simulink model "reference_generator"  (Simulink 8.2)
settings: Solver=FixedStepDiscrete  StartTime=0.0  StopTime=60  FixedStep=0.1  RelTol=1e-3
undefined symbols (not defined in the file or in its folder): sigbuilder_block
settings Model: Creator=ovidiua  LastModifiedBy=ovidiua
settings DataIOCC: SignalLoggingSaveFormat=Dataset
settings OptimizationCC: ExpressionDepthLimit=128
settings DebuggingCC: FcnCallInpInsideContextMsg=EnableAllAsError  StateNameClashWarn=none
settings GRTTargetCC: CombineOutputUpdateFcns=on  GRTInterface=off

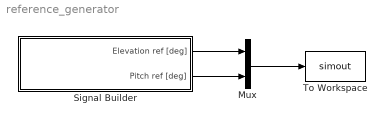
== system reference_generator ==
  Mux : Mux  Inputs=2
  Signal Builder : Subsystem  Tag=STV Subsys  LoadFcn=sigbuilder_block('load');  StartFcn=sigbuilder_block('start');  StopFcn=sigbuilder_block('stop');  ClipboardFcn=sigbuilder_block('clipboard');  mask(Sigbuilder block){}
      mask help: Simulink:masks:SigbuilderBlock_MD
      mask init:
      | if ~strcmp(get_param(bdroot(gcbh),'SimulationStatus'),'stopped') tuvar = sigbuilder_block('maskInit'); end
      settings: CopyFcn=sigbuilder_block('copy');  DeleteFcn=sigbuilder_block('delete');  ModelCloseFcn=sigbuilder_block('modelClose');  PreSaveFcn=sigbuilder_block('preSave');  PauseFcn=sigbuilder_block('pause');  ContinueFcn=sigbuilder_block('continue');  NameChangeFcn=sigbuilder_block('namechange');  OpenFcn=sigbuilder_block('open',[446.25 160.5 761.25 513.75 ]);  CloseFcn=sigbuilder_block('close');
      mask Display: plot(0, 0, 100, 100,[2, 2, 32, 32, 2], [68, 8, 8, 68, 68],[32, 2], [38, 38], [32, 19, 2],[53, 60, 44], [32, 17, 17, 2],[16, 16, 31, 31]);txt = getActiveGroup(gcbh);text(2, 100, txt,'verticalAlignment', 'top');
  To Workspace : ToWorkspace  VariableName=simout  SampleTime=-1  SaveFormat=Timeseries
  wires:
  Signal Builder/1(Elevation ref [deg]) -> Mux/1
  Signal Builder/2(Pitch ref [deg]) -> Mux/2
  Mux/1 -> To Workspace/1

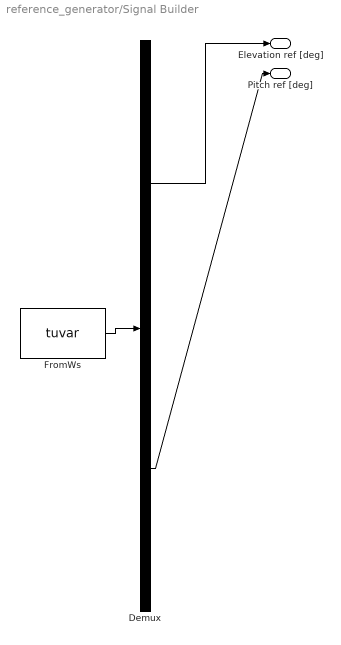
== system reference_generator/Signal Builder ==
  Demux : Demux  Tag=STV Demux  Outputs=2
  FromWs : FromWorkspace  Tag=STV FromWs  VariableName=tuvar  SampleTime=0  SigBuilderData=DataTag0  VnvData=DataTag1
      SigBuilderData=|
      | common.afterFinalStr = 'Extrapolate'
      | common.sampleTime = 0
      | dataSet.timeRange = [0 60]
      | dataSet.name = 'Group 1'
      | sbobj.Groups.Name = 'Group 1'
      | sbobj.Groups.Signals(1).Name = 'Elevation ref [deg]'
      | sbobj.Groups.Signals(1).XData = [0 10 15 40 45 50 55 60]
      | sbobj.Groups.Signals(1).YData = [0 0 25.1497487437 25 0 -15 0 0]
      | sbobj.Groups.Signals(2).Name = 'Pitch ref [deg]'
      | sbobj.Groups.Signals(2).XData = [0 20 23 30 34 34 35 60]
      | sbobj.Groups.Signals(2).YData = [0 0 30 30 -30 -29.5 0 0]
      | sbobj.Groups.TimeRange = [0 60]
  Elevation ref [deg] : Outport  Tag=STV Outport
  Pitch ref [deg] : Outport  Tag=STV Outport  Port=2
  wires:
  Demux/1 -> Elevation ref [deg]/1
  FromWs/1 -> Demux/1
  Demux/2 -> Pitch ref [deg]/1
